simulink model "walkingRobot"  (R2020a)
settings: Solver=ode15s  StartTime=0.0  StopTime=10  EnableMultiTasking=on
PreLoadFcn:
  | robotParameters
  | load('defaultsimulationinputs.mat')
undefined symbols (not defined in the file or in its folder): ankle_servo_kd, ankle_servo_ki, ankle_servo_kp, deriv_filter_coeff, hip_servo_kd, hip_servo_ki, hip_servo_kp, init_angs_L, init_angs_R, knee_servo_kd, knee_servo_ki, knee_servo_kp, max_torque, motion_time_constant
libraries: simulink x13, simulink_extras x12, walkingRobotUtils x5
(part 2 of 2)

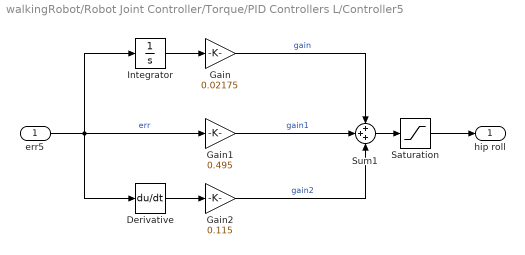
== system walkingRobot/Robot Joint Controller/Torque/PID Controllers L/Controller5 ==
  err5 : Inport
  Derivative : Derivative
  Gain : Gain  Gain=0.02175
  Gain1 : Gain  Gain=0.495
  Gain2 : Gain  Gain=0.115
  Integrator : Integrator
  Saturation : Saturate  UpperLimit=15  LowerLimit=-15
  Sum1 : Sum  Inputs=+++
  hip roll : Outport
  wires:
  Gain/1 -> Sum1/1  "gain"
  Saturation/1 -> hip roll/1
  Gain1/1 -> Sum1/2  "gain1"
  Gain2/1 -> Sum1/3  "gain2"
  err5/1 -> Derivative/1, Gain1/1, Integrator/1  "err"
  Derivative/1 -> Gain2/1
  Sum1/1 -> Saturation/1
  Integrator/1 -> Gain/1

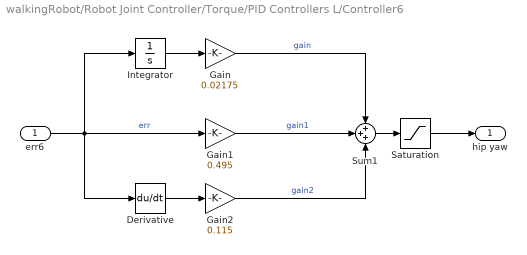
== system walkingRobot/Robot Joint Controller/Torque/PID Controllers L/Controller6 ==
  err6 : Inport
  Derivative : Derivative
  Gain : Gain  Gain=0.02175
  Gain1 : Gain  Gain=0.495
  Gain2 : Gain  Gain=0.115
  Integrator : Integrator
  Saturation : Saturate  UpperLimit=15  LowerLimit=-15
  Sum1 : Sum  Inputs=+++
  hip yaw : Outport
  wires:
  Gain/1 -> Sum1/1  "gain"
  Saturation/1 -> hip yaw/1
  Gain1/1 -> Sum1/2  "gain1"
  Gain2/1 -> Sum1/3  "gain2"
  err6/1 -> Derivative/1, Gain1/1, Integrator/1  "err"
  Derivative/1 -> Gain2/1
  Sum1/1 -> Saturation/1
  Integrator/1 -> Gain/1

== system walkingRobot/Robot Joint Controller/Torque/PID Controllers R/Controller ==
  err1 : Inport
  Derivative : Derivative
  Gain1 : Gain  Gain=0.02175
  Gain2 : Gain  Gain=0.495
  Gain3 : Gain  Gain=0.115
  Integrator : Integrator
  Saturation : Saturate  UpperLimit=15  LowerLimit=-15
  Sum1 : Sum  Inputs=+++
  ankle roll : Outport
  wires:
  Gain1/1 -> Sum1/1  "gain1"
  Saturation/1 -> ankle roll/1
  Gain2/1 -> Sum1/2  "gain2"
  Gain3/1 -> Sum1/3  "gain3"
  err1/1 -> Derivative/1, Gain2/1, Integrator/1  "err"
  Derivative/1 -> Gain3/1
  Sum1/1 -> Saturation/1
  Integrator/1 -> Gain1/1

== system walkingRobot/Robot Joint Controller/Torque/PID Controllers R/Controller1 ==
  err2 : Inport
  Derivative : Derivative
  Gain4 : Gain  Gain=0.02175
  Gain5 : Gain  Gain=0.495
  Gain6 : Gain  Gain=0.115
  Integrator : Integrator
  Saturation : Saturate  UpperLimit=15  LowerLimit=-15
  Sum1 : Sum  Inputs=+++
  ankle pitch : Outport
  wires:
  Gain4/1 -> Sum1/1  "gain4"
  Saturation/1 -> ankle pitch/1
  Gain5/1 -> Sum1/2  "gain5"
  Gain6/1 -> Sum1/3  "gain6"
  err2/1 -> Derivative/1, Gain5/1, Integrator/1  "err"
  Derivative/1 -> Gain6/1
  Sum1/1 -> Saturation/1
  Integrator/1 -> Gain4/1

== system walkingRobot/Robot Joint Controller/Torque/PID Controllers R/Controller2 ==
  err3 : Inport
  Derivative : Derivative
  Gain7 : Gain  Gain=0.02175
  Gain8 : Gain  Gain=0.495
  Gain9 : Gain  Gain=0.115
  Integrator : Integrator
  Saturation : Saturate  UpperLimit=15  LowerLimit=-15
  Sum1 : Sum  Inputs=+++
  knee : Outport
  wires:
  Gain7/1 -> Sum1/1  "gain7"
  Saturation/1 -> knee/1
  Gain8/1 -> Sum1/2  "gain8"
  Gain9/1 -> Sum1/3  "gain9"
  err3/1 -> Derivative/1, Gain8/1, Integrator/1  "err"
  Derivative/1 -> Gain9/1
  Sum1/1 -> Saturation/1
  Integrator/1 -> Gain7/1

== system walkingRobot/Robot Joint Controller/Torque/PID Controllers R/Controller3 ==
  err4 : Inport
  Derivative : Derivative
  Gain10 : Gain  Gain=0.02175
  Gain11 : Gain  Gain=0.495
  Gain12 : Gain  Gain=0.115
  Integrator : Integrator
  Saturation : Saturate  UpperLimit=15  LowerLimit=-15
  Sum1 : Sum  Inputs=+++
  hip pitch : Outport
  wires:
  Gain10/1 -> Sum1/1  "gain10"
  Saturation/1 -> hip pitch/1
  Gain11/1 -> Sum1/2  "gain11"
  Gain12/1 -> Sum1/3  "gain12"
  err4/1 -> Derivative/1, Gain11/1, Integrator/1  "err"
  Derivative/1 -> Gain12/1
  Sum1/1 -> Saturation/1
  Integrator/1 -> Gain10/1

== system walkingRobot/Robot Joint Controller/Torque/PID Controllers R/Controller4 ==
  err5 : Inport
  Derivative : Derivative
  Gain13 : Gain  Gain=0.02175
  Gain14 : Gain  Gain=0.495
  Gain15 : Gain  Gain=0.115
  Integrator : Integrator
  Saturation : Saturate  UpperLimit=15  LowerLimit=-15
  Sum1 : Sum  Inputs=+++
  hip roll : Outport
  wires:
  Gain13/1 -> Sum1/1  "gain13"
  Saturation/1 -> hip roll/1
  Gain14/1 -> Sum1/2  "gain14"
  Gain15/1 -> Sum1/3  "gain15"
  err5/1 -> Derivative/1, Gain14/1, Integrator/1  "err"
  Derivative/1 -> Gain15/1
  Sum1/1 -> Saturation/1
  Integrator/1 -> Gain13/1

== system walkingRobot/Robot Joint Controller/Torque/PID Controllers R/Controller5 ==
  err6 : Inport
  Derivative : Derivative
  Gain16 : Gain  Gain=0.02175
  Gain17 : Gain  Gain=0.495
  Gain18 : Gain  Gain=0.115
  Integrator : Integrator
  Saturation : Saturate  UpperLimit=15  LowerLimit=-15
  Sum1 : Sum  Inputs=+++
  hip yaw : Outport
  wires:
  Gain16/1 -> Sum1/1  "gain16"
  Saturation/1 -> hip yaw/1
  Gain17/1 -> Sum1/2  "gain17"
  Gain18/1 -> Sum1/3  "gain18"
  err6/1 -> Derivative/1, Gain17/1, Integrator/1  "err"
  Derivative/1 -> Gain18/1
  Sum1/1 -> Saturation/1
  Integrator/1 -> Gain16/1

== matlab function walkingRobot/Inverse Kinematics/Inverse Kinematics R ==
  data: transmat input; q output; isLeft input
function q = inverseKinematics(transmat, isLeft)
q = invKinBody2Foot(transmat, isLeft);

== matlab function walkingRobot/Inverse Kinematics/Inverse Kinematics L ==
  data: transmat input; q output; isLeft input
function q = inverseKinematics(transmat, isLeft)
q = invKinBody2Foot(transmat, isLeft);
